simulink model "likestromsmotor2"  (R2017b)
settings: Solver=VariableStepAuto  StartTime=0.0  StopTime=simtime  RelTol=1e-3
values from neighbouring files (symbols this model uses):
  K = 1/(4*T1)    (= 3.90625)    [oppg2.m]    (also in oppg3.m = input(' K :'))
  T1 = 0.064    [oppg2.m]    (also in oppg3.m = 4)
  T2 = 0.01    [oppg2.m]    (also in oppg3.m = 1.5)
  y0 = 1    [oppg2.m]
settings Model: Creator=bendi  LastModifiedBy=bruker

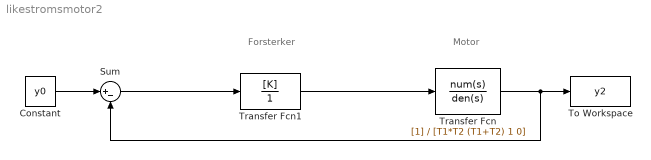
== system likestromsmotor2 ==
  note: Motor
  note: Forsterker
  Constant : Constant  Value=y0
  Sum : Sum  Inputs=|+-
  To Workspace : ToWorkspace  VariableName=y2  SaveFormat=Timeseries  SampleTime=-1
  Transfer Fcn : TransferFcn  Denominator=[T1*T2 (T1+T2) 1 0]
  Transfer Fcn1 : TransferFcn  Numerator=[K]  Denominator=1
  wires:
  Sum/1 -> Transfer Fcn1/1
  Constant/1 -> Sum/1
  Transfer Fcn1/1 -> Transfer Fcn/1
  Transfer Fcn/1 -> Sum/2, To Workspace/1
